simulink model "dspsinecomp_frame"  (Simulink 8.3)
settings: Solver=FixedStepDiscrete  StartTime=0.0  StopTime=inf  RelTol=1e-3
libraries: dspstat3 x4, dspsrcs4 x3, dspmisc x1
Description:
  | Comparison of frame-based sine wave generation techniques.
CloseFcn:
  | clear y1;
  | clear y2;
  | clear y3;
settings Model: Creator=The MathWorks Inc.  ExtModeTrigMode=oneshot  ExtModeArmWhenConnect=off
settings DataIOCC: LimitDataPoints=off  SaveOutput=off  SaveTime=off
settings OptimizationCC: BlockReduction=off  BooleanDataType=off  ExpressionDepthLimit=2147483647  RollThreshold=2  InitFltsAndDblsToZero=on
settings DebuggingCC: SaveWithParameterizedLinksMsg=none  SignalResolutionControl=TryResolveAllWithWarning  SolverPrmCheckMsg=none  MultiTaskDSMMsg=warning  MultiTaskCondExecSysMsg=none  IntegerOverflowMsg=none  FcnCallInpInsideContextMsg=UseLocalSettings  StrictBusMsg=None
settings HardwareCC: TargetUnknown=on
settings RTWCC: IncludeERTFirstTime=on
settings GRTTargetCC: TargetFcnLib=ansi_tfl_tmw.mat

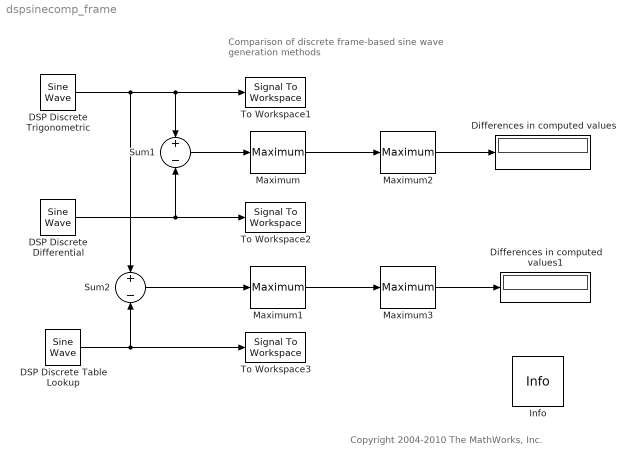
== system dspsinecomp_frame ==
  note: Comparison of discrete frame-based
      | sine wave generation methods
  note: Copyright 2004-2010 The MathWorks, Inc.
  DSP Discrete Differential : dspsrcs4/Sine Wave  Amplitude=1  Frequency=1e4  Phase=0  SampleMode=Discrete  OutComplex=Real  CompMethod=Differential  TableSize=Speed  SampleTime=1e-5  SamplesPerFrame=32  ResetState=Restart at time zero  dataType=double  wordLen=16  udDataType=sfix(16)  fracBitsMode=Best precision  numFracBits=15  OutDataTypeStr=double  LastOutDataTypeStr=double
  DSP Discrete Table Lookup : dspsrcs4/Sine Wave  Amplitude=1  Frequency=1e4  Phase=0  SampleMode=Discrete  OutComplex=Real  CompMethod=Table lookup  TableSize=Speed  SampleTime=1e-5  SamplesPerFrame=32  ResetState=Restart at time zero  dataType=double  wordLen=16  udDataType=sfix(16)  fracBitsMode=Best precision  numFracBits=15  OutDataTypeStr=double  LastOutDataTypeStr=double
  DSP Discrete Trigonometric : dspsrcs4/Sine Wave  Amplitude=1  Frequency=1e4  Phase=0  SampleMode=Discrete  OutComplex=Real  CompMethod=Trigonometric fcn  TableSize=Speed  SampleTime=1e-5  SamplesPerFrame=32  ResetState=Restart at time zero  dataType=double  wordLen=16  udDataType=sfix(16)  fracBitsMode=Best precision  numFracBits=15  OutDataTypeStr=double  LastOutDataTypeStr=double
  Differences in computed values : Display
  Differences in computed values1 : Display
  Info : dspmisc/Info  SystemSampleTime=-1
  Maximum : dspstat3/Maximum  fcn=Running  reset=None  InputProcessing=Columns as channels (frame based)  indexBase=One  operateOver=Each column  Dimension=1  colComp=on  operation=maximum  roiEnable=off  roiType=Rectangles  roiPortion=Entire ROI  roiOutput=Individual statistics for each ROI  roiFlag=off  accumDataTypeStr=Inherit: Same as product output  accumLastDataTypeStr=Inherit: Same as product output  roundingMode=Floor  overflowMode=off
  Maximum1 : dspstat3/Maximum  fcn=Running  reset=None  InputProcessing=Columns as channels (frame based)  indexBase=One  operateOver=Each column  Dimension=1  colComp=on  operation=maximum  roiEnable=off  roiType=Rectangles  roiPortion=Entire ROI  roiOutput=Individual statistics for each ROI  roiFlag=off  accumDataTypeStr=Inherit: Same as product output  accumLastDataTypeStr=Inherit: Same as product output  roundingMode=Floor  overflowMode=off
  Maximum2 : dspstat3/Maximum  fcn=Value  reset=None  InputProcessing=Columns as channels (frame based)  indexBase=One  operateOver=Each column  Dimension=1  colComp=on  operation=maximum  roiEnable=off  roiType=Rectangles  roiPortion=Entire ROI  roiOutput=Individual statistics for each ROI  roiFlag=off  accumDataTypeStr=Inherit: Same as product output  accumLastDataTypeStr=Inherit: Same as product output  roundingMode=Floor  overflowMode=off
  Maximum3 : dspstat3/Maximum  fcn=Value  reset=None  InputProcessing=Columns as channels (frame based)  indexBase=One  operateOver=Each column  Dimension=1  colComp=on  operation=maximum  roiEnable=off  roiType=Rectangles  roiPortion=Entire ROI  roiOutput=Individual statistics for each ROI  roiFlag=off  accumDataTypeStr=Inherit: Same as product output  accumLastDataTypeStr=Inherit: Same as product output  roundingMode=Floor  overflowMode=off
  Sum1 : Sum  Inputs=+-  SaturateOnIntegerOverflow=on  InputSameDT=on  OutDataTypeStr=Inherit: Same as first input
  Sum2 : Sum  Inputs=+-  SaturateOnIntegerOverflow=on  InputSameDT=on  OutDataTypeStr=Inherit: Same as first input
  To Workspace1 : SignalToWorkspace  VariableName=y1
  To Workspace2 : SignalToWorkspace  VariableName=y2
  To Workspace3 : SignalToWorkspace  VariableName=y3
  wires:
  DSP Discrete Trigonometric/1 -> Sum1/1, To Workspace1/1, Sum2/1
  Sum1/1 -> Maximum/1
  Maximum/1 -> Maximum2/1
  DSP Discrete Differential/1 -> Sum1/2, To Workspace2/1
  Sum2/1 -> Maximum1/1
  DSP Discrete Table Lookup/1 -> Sum2/2, To Workspace3/1
  Maximum1/1 -> Maximum3/1
  Maximum2/1 -> Differences in computed values/1
  Maximum3/1 -> Differences in computed values1/1
